simulink model "Model_Dimitri"  (R2023b)
settings: Solver=ode23tb  StartTime=0.0  StopTime=1.5  FixedStep=1e-6  MaxStep=1/50/100  RelTol=1e-3
values from neighbouring files (symbols this model uses):
  B = 0.0129    [PARAMETERS_MODEL_GR2.m]    (also in Parameters.m; Parameters_Chloe.m)
  C_dc = 15e-3    (= 0.015)    [PARAMETERS_MODEL_GR2.m]    (also in Parameters.m; Parameters_Chloe.m)
  f_grid = 50    [PARAMETERS_MODEL_GR2.m]    (also in Parameters.m; Parameters_Chloe.m)
  f_r = 50    [PARAMETERS_MODEL_GR2.m]    (also in Parameters.m; Parameters_Chloe.m)
  J = 0.2799    [PARAMETERS_MODEL_GR2.m]    (also in Parameters.m; Parameters_Chloe.m)
  L_grid = 1.5e-6    (= 1.5e-06)    [PARAMETERS_MODEL_GR2.m]    (also in Parameters.m = 1e-12; Parameters_Chloe.m = 2e-05)
  L_lr = 1.8e-3    (= 0.0018)    [PARAMETERS_MODEL_GR2.m]    (also in Parameters.m = 1.8; Parameters_Chloe.m)
  L_ls = 1.8e-3    (= 0.0018)    [PARAMETERS_MODEL_GR2.m]    (also in Parameters.m = 1.8; Parameters_Chloe.m)
  L_rectif = 10e-3    (= 0.01)    [PARAMETERS_MODEL_GR2.m]    (also in Parameters.m; Parameters_Chloe.m)
  P = 4    [PARAMETERS_MODEL_GR2.m]    (also in Parameters.m; Parameters_Chloe.m)
  P_r = 19e3    (= 19000)    [PARAMETERS_MODEL_GR2.m]    (also in Parameters.m; Parameters_Chloe.m)
  R_grid = 0.005    [PARAMETERS_MODEL_GR2.m]    (also in Parameters.m = 0.001; Parameters_Chloe.m = 0.2)
  R_r = 0.1091    [PARAMETERS_MODEL_GR2.m]    (also in Parameters.m; Parameters_Chloe.m)
  R_s = 0.0629    [PARAMETERS_MODEL_GR2.m]    (also in Parameters.m; Parameters_Chloe.m)
  U_ac = 380    [PARAMETERS_MODEL_GR2.m]    (also in Parameters.m; Parameters_Chloe.m)
  V_r = 400    [PARAMETERS_MODEL_GR2.m]    (also in Parameters.m; Parameters_Chloe.m)
libraries: spsSeriesRLCBranchLib x10, spsDiodeLib x6, spsMosfetLib x6, spsVoltageMeasurementLib x5, spsThreePhaseVIMeasurementLib x4, spsACVoltageSourceLib x3, spsThreePhaseTransformerTwoWindingsLib x2, spsAsynchronousMachinepuUnitsLib x2, spsCurrentMeasurementLib x2, spsGroundLib x1, spsThreePhaseSourceLib x1, spsTriangleGeneratorLib x1
settings Model: Creator=dimit  LastModifiedBy=dimit

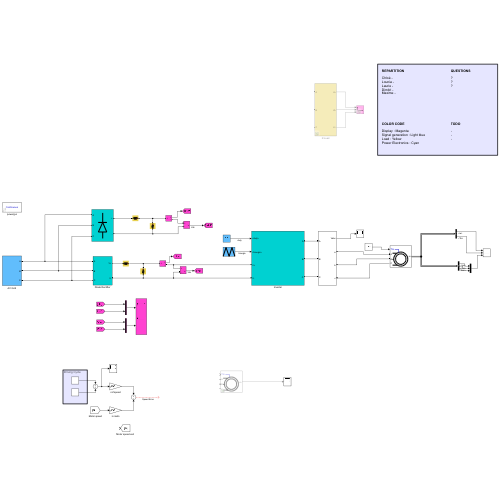
[thumbnail: Simulink's stored preview of the top-level diagram]
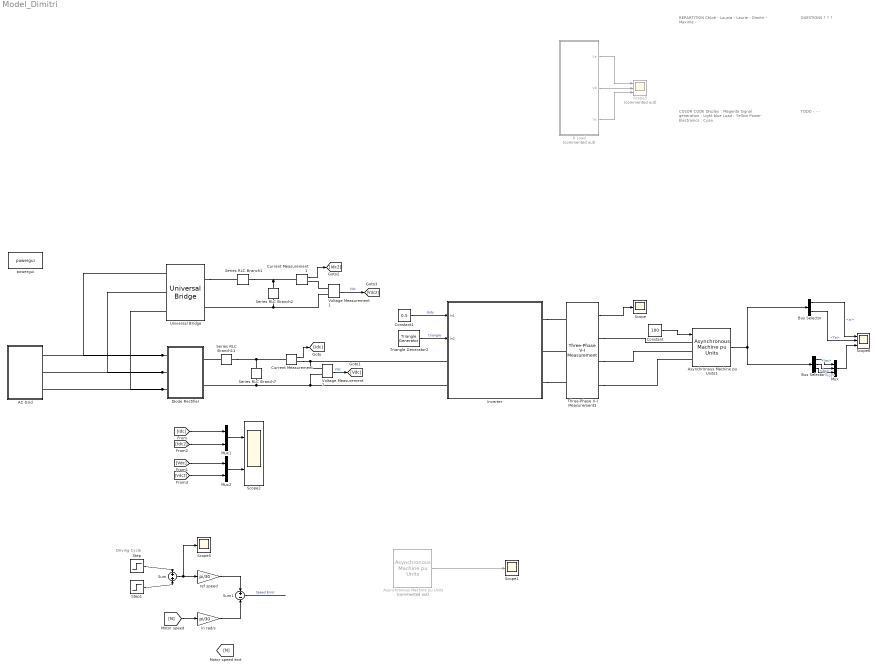
== system Model_Dimitri ==
  note: COLOR CODE
      |
      | Display : Magenta
      | Signal generation : Light blue
      | Load : Yellow
      | Power Electronics : Cyan
  note: Driving Cycle
  note: QUESTIONS
      |
      | ?
      | ?
      | ?
  note: TODO
      |
      | -
      | -
      | -
  note: REPARTITION
      |
      | Chloé -
      | Lounia -
      | Laurie -
      | Dimitri -
      | Maxime -
  AC Grid : Subsystem
  Asynchronous Machine pu Units : spsAsynchronousMachinepuUnitsLib/Asynchronous Machine pu Units  Commented=on  RotorType=Squirrel-cage  PresetModel=No  MechanicalLoad=Torque Tm  ShowDetailedParameters=on  ReferenceFrame=Rotor  Units=pu  MeasurementBus=on  NominalParameters=[3730 460 60]  VoltageRatio=1  Stator=[R_s L_ls]  Rotor=[R_r L_lr]  Cage1=[0.01909 0.0397]  Cage2=[0.01909 0.0397]  Lm=L_m  Mechanical=[J B P]  PolePairs=2  InitialConditions="[ 1,0   0,0,0   0,0,0 ]"  SimulateSaturation=off  Saturation="[0.212,0.4201,0.8125,1.0979,1.4799,2.2457,3.2586,4.5763,6.4763 ;   0.5,0.7,0.9,1,1.1,1.2 ,1.3,1.4,1.5]"  LoadFlowParameters=0  TsPowergui=0  TsBlock=-1  IterativeModel=Trapezoidal non iterative  IterativeDiscreteModel=Trapezoidal non iterative  Pmec=0
      settings: LibrarySourceBlock=|
      | sps_lib/Electrical Machines/Asynchronous Machine
      | pu Units
  Asynchronous Machine pu Units1 : spsAsynchronousMachinepuUnitsLib/Asynchronous Machine pu Units  RotorType=Squirrel-cage  PresetModel=No  MechanicalLoad=Torque Tm  ShowDetailedParameters=on  ReferenceFrame=Rotor  Units=pu  MeasurementBus=on  NominalParameters=[P_r V_r f_r]  VoltageRatio=1  Stator=[R_s L_ls]  Rotor=[R_r L_lr]  Cage1=[0.01909 0.0397]  Cage2=[0.01909 0.0397]  Lm=L_m  Mechanical=[J B P]  PolePairs=2  InitialConditions="[ 1,0   0,0,0   0,0,0]"  SimulateSaturation=off  Saturation="[0.212,0.4201,0.8125,1.0979,1.4799,2.2457,3.2586,4.5763,6.4763 ;   0.5,0.7,0.9,1,1.1,1.2 ,1.3,1.4,1.5]"  LoadFlowParameters=0  TsPowergui=0  TsBlock=-1  IterativeModel=Trapezoidal non iterative  IterativeDiscreteModel=Trapezoidal non iterative  Pmec=0
      settings: LibrarySourceBlock=|
      | sps_lib/Electrical Machines/Asynchronous Machine
      | pu Units
  Bus Selector : BusSelector  OutputSignals=w,Te
  Bus Selector1 : BusSelector  OutputSignals=ias,ibs,ics
  Constant : Constant  Value=100
  Constant1 : Constant  Value=0.5
  Current Measurement : spsCurrentMeasurementLib/Current Measurement  PhasorSimulation=off  OutputType=Complex  PSBequivalent=0
  Current Measurement1 : spsCurrentMeasurementLib/Current Measurement  PhasorSimulation=off  OutputType=Complex  PSBequivalent=0
  Diode Rectifier : Subsystem
  Inverter : Subsystem
  Mux : Mux  Inputs=3
  Mux1 : Mux  Inputs=2
  Mux2 : Mux  Inputs=2
  R Load : Subsystem  Commented=on
  Scope : Scope
  Scope1 : Scope
  Scope2 : Scope  NumInputPorts=2
  Scope3 : Scope  Commented=on  NumInputPorts=3
  Scope5 : Scope
  Scope6 : Scope  NumInputPorts=3
  Series RLC Branch1 : spsSeriesRLCBranchLib/Series RLC Branch  LConnTagsString=__new0  RConnTagsString=__new0  BranchType=L  Resistance=1  Inductance=L_rectif  SetiL0=off  InitialCurrent=0  Capacitance=15e-6  Setx0=off  InitialVoltage=0  Measurements=None
  Series RLC Branch11 : spsSeriesRLCBranchLib/Series RLC Branch  LConnTagsString=__new0  RConnTagsString=__new0  BranchType=L  Resistance=1  Inductance=L_rectif  SetiL0=off  InitialCurrent=0  Capacitance=15e-6  Setx0=off  InitialVoltage=0  Measurements=None
  Series RLC Branch2 : spsSeriesRLCBranchLib/Series RLC Branch  LConnTagsString=__new0  RConnTagsString=__new0  BranchType=C  Resistance=1  Inductance=1e-3  SetiL0=off  InitialCurrent=0  Capacitance=C_dc  Setx0=off  InitialVoltage=0  Measurements=None
  Series RLC Branch7 : spsSeriesRLCBranchLib/Series RLC Branch  LConnTagsString=__new0  RConnTagsString=__new0  BranchType=C  Resistance=1  Inductance=1e-3  SetiL0=off  InitialCurrent=0  Capacitance=C_dc  Setx0=off  InitialVoltage=0  Measurements=None
  Step : Step  Time=0.1  After=1200  SampleTime=0
  Step1 : Step  Time=1.7  After=-1200  SampleTime=0
  Sum : Sum  Inputs=+|+
  Sum1 : Sum  Inputs=+|-
  Three-Phase V-I Measurement1 : spsThreePhaseVIMeasurementLib/Three-Phase V-I Measurement  VoltageMeasurement=phase-to-phase  SetLabelV=off  LabelV=Vabc  Vpu=off  VpuLL=off  CurrentMeasurement=no  SetLabelI=off  LabelI=Iabc  Ipu=off  Pbase=100e6  Vbase=500e3  OutputType=Complex  PhasorSimulation=off  PSBequivalent=0
  Triangle Generator2 : spsTriangleGeneratorLib/Triangle Generator  Freq=f_r*39  Phase=0  Ts=0
  Universal Bridge : spsUniversalBridgeLib/Universal Bridge  Arms=3  SnubberResistance=R_snubber  SnubberCapacitance=C_snubber  Device=Diodes  Ron=R_on  Lon=0  ForwardVoltages="[  0  0  ]"  ForwardVoltage=V_f  GTOparameters=[ 10e-6 , 20e-6 ]  IGBTparameters=[ 1e-6 , 2e-6 ]  Measurements=None  Measurements_2=None  converterType=Rectifier
  Voltage Measurement1 : spsVoltageMeasurementLib/Voltage Measurement  PhasorSimulation=off  OutputType=Complex  PSBequivalent=0
  Voltage Measurement7 : spsVoltageMeasurementLib/Voltage Measurement  PhasorSimulation=off  OutputType=Complex  PSBequivalent=0
  in rad/s : Gain  Gain=pi/30
  powergui : sps_lib/powergui  Priority=1  SimulationMode=Continuous  SampleTime=1e-6  frequency=60  Iterations=50  frequencyindice=50  Pbase=100e6  ErrMax=1e-4  UnitsV=kV  UnitsW=MW  buscounter=0  FunctionMessages=off  echomessages=off  EnableUseOfTLC=off  CurrentSourceSwitches=off  DisableSnubberDevices=off  DisableRonSwitches=off  DisableVfSwitches=off  DisplayEquations=off  AutomaticDiscreteSolvers=off  SolverType=Tustin/Backward Euler (TBE)  Interpol=off  ExternalGateDelay=off  methode=off  Ts=100  x0status=blocks  SPID=on  SwTol=0  HookPort=off  NonlinearTolerance=1e-4  nMaxIteration=100  ContinueOnMaxIteration=off  RestoreLinks=warning  ResistiveCurrentMeasurement=off  Frange=[0:2:500]  Ylog=off  Xlog=on  ShowGrid=off  save=off  variable=ZData  structure=0  ZoomFFT=off  StartTime=0.0  cycles=1  DisplayStyle=1  fundamental=60  FreqAxis=off  MaxFrequency=1000  frequencyindicesteady=1  RmsSteady=1  display=off
  ref speed : Gain  Gain=pi/30
  wires:
  Triangle Generator2/1 -> Inverter/2(In2)  "triangle"
  Constant1/1 -> Inverter/1(In1)  "duty"
  Sum1/1 -> ?  "Speed Error"
  [N] -> in rad/s/1
  Step1/1 -> Sum/2
  Sum/1 -> ref speed/1, Scope5/1
  ref speed/1 -> Sum1/1
  in rad/s/1 -> Sum1/2
  Step/1 -> Sum/1
  Asynchronous Machine pu Units/1 -> Scope1/1
  R Load/1(Va) -> Scope3/1
  R Load/2(Vb) -> Scope3/2
  R Load/3(Vc) -> Scope3/3
  Constant/1 -> Asynchronous Machine pu Units1/1
  Asynchronous Machine pu Units1/1 -> Bus Selector/1, Bus Selector1/1
  Bus Selector1/1 -> Mux/1  "<ias>"
  Bus Selector1/2 -> Mux/2  "<ibs>"
  Bus Selector1/3 -> Mux/3  "<ics>"
  Mux/1 -> Scope6/3
  Bus Selector/1 -> Scope6/1  "<w>"
  Bus Selector/2 -> Scope6/2  "<Te>"
  Three-Phase V-I Measurement1/1 -> Scope/1
  Current Measurement/1 -> [Idc]
  Voltage Measurement7/1 -> [Vdc]  "Vdc"
  Current Measurement1/1 -> [Idc2]
  Voltage Measurement1/1 -> [Vdc2]  "Vdc"
  [Idc] -> Mux1/1
  [Vdc] -> Mux2/1
  [Vdc2] -> Mux2/2
  [Idc2] -> Mux1/2
  Mux1/1 -> Scope2/1
  Mux2/1 -> Scope2/2
  connections:
  Diode Rectifier/LConn1 -- Universal Bridge/LConn1 -- AC Grid/LConn1
  Diode Rectifier/LConn2 -- Universal Bridge/LConn2 -- AC Grid/LConn2
  Diode Rectifier/LConn3 -- Universal Bridge/LConn3 -- AC Grid/LConn3
  Inverter/LConn2 -- Diode Rectifier/RConn2 -- Series RLC Branch7/RConn1 -- Voltage Measurement7/LConn2
  Voltage Measurement7/LConn1 -- Inverter/LConn1 -- Current Measurement/RConn1
  Series RLC Branch11/RConn1 -- Diode Rectifier/RConn1
  Series RLC Branch11/LConn1 -- Current Measurement/LConn1 -- Series RLC Branch7/LConn1
  Three-Phase V-I Measurement1/LConn2 -- Inverter/RConn2
  Inverter/RConn1 -- Three-Phase V-I Measurement1/LConn1
  Inverter/RConn3 -- Three-Phase V-I Measurement1/LConn3
  Three-Phase V-I Measurement1/RConn1 -- Asynchronous Machine pu Units1/LConn1
  Three-Phase V-I Measurement1/RConn2 -- Asynchronous Machine pu Units1/LConn2
  Three-Phase V-I Measurement1/RConn3 -- Asynchronous Machine pu Units1/LConn3
  Voltage Measurement1/LConn1 -- Current Measurement1/RConn1
  Series RLC Branch2/LConn1 -- Series RLC Branch1/LConn1 -- Current Measurement1/LConn1
  Series RLC Branch2/RConn1 -- Voltage Measurement1/LConn2 -- Universal Bridge/RConn2
  Universal Bridge/RConn1 -- Series RLC Branch1/RConn1

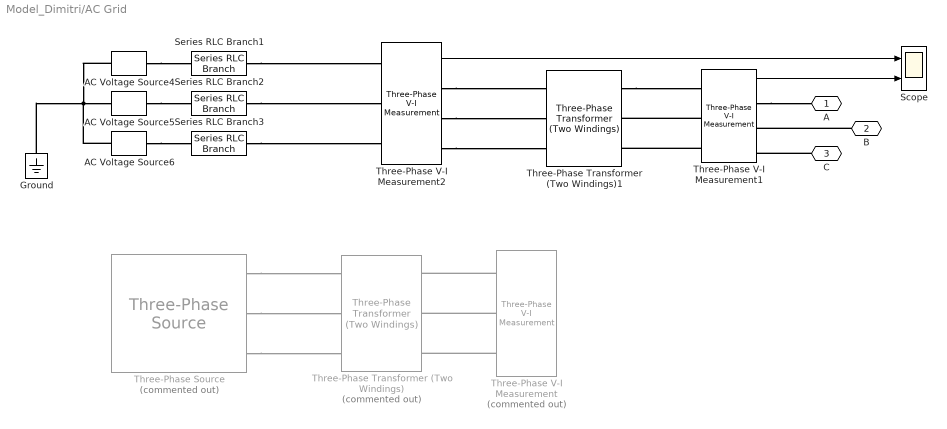
== system Model_Dimitri/AC Grid ==
  AC Voltage Source4 : spsACVoltageSourceLib/AC Voltage Source  Amplitude=U_ac/sqrt(3)*sqrt(2)  Phase=0  Frequency=f_grid  SampleTime=0  Measurements=None  BusType=swing  Pref=10e3  Qref=0  Qmin=-inf  Qmax=+inf
  AC Voltage Source5 : spsACVoltageSourceLib/AC Voltage Source  Amplitude=U_ac/sqrt(3)*sqrt(2)  Phase=-120  Frequency=f_grid  SampleTime=0  Measurements=None  BusType=swing  Pref=10e3  Qref=0  Qmin=-inf  Qmax=+inf
  AC Voltage Source6 : spsACVoltageSourceLib/AC Voltage Source  Amplitude=U_ac/sqrt(3)*sqrt(2)  Phase=120  Frequency=f_grid  SampleTime=0  Measurements=None  BusType=swing  Pref=10e3  Qref=0  Qmin=-inf  Qmax=+inf
  Ground : spsGroundLib/Ground  LConnTagsString=a
  Scope : Scope  NumInputPorts=2
  Series RLC Branch1 : spsSeriesRLCBranchLib/Series RLC Branch  LConnTagsString=__new0  RConnTagsString=__new0  BranchType=RL  Resistance=R_grid  Inductance=L_grid  SetiL0=off  InitialCurrent=0  Capacitance=15e-6  Setx0=off  InitialVoltage=0  Measurements=None
  Series RLC Branch2 : spsSeriesRLCBranchLib/Series RLC Branch  LConnTagsString=__new0  RConnTagsString=__new0  BranchType=RL  Resistance=R_grid  Inductance=L_grid  SetiL0=off  InitialCurrent=0  Capacitance=15e-6  Setx0=off  InitialVoltage=0  Measurements=None
  Series RLC Branch3 : spsSeriesRLCBranchLib/Series RLC Branch  LConnTagsString=__new0  RConnTagsString=__new0  BranchType=RL  Resistance=R_grid  Inductance=L_grid  SetiL0=off  InitialCurrent=0  Capacitance=15e-6  Setx0=off  InitialVoltage=0  Measurements=None
  Three-Phase Transformer (Two Windings) : spsThreePhaseTransformerTwoWindingsLib/Three-Phase Transformer (Two Windings)  Commented=on  Winding1Connection=Y  Winding2Connection=Y  CoreType=Three single-phase transformers  SetSaturation=off  Hysteresis=off  DataFile='hysteresis'  SetInitialFlux=off  Measurements=None  UNITS=pu  NominalPower=[ 20e3 , 50 ]  Winding1=[ 380 , 0.002 , 0.08 ]  Winding2=[ 380 , 0.002 , 0.08 ]  Rm=500  Lm=500  L0=0.5  Saturation=[ 0,0 ; 0.0024,1.2 ; 1.0,1.52 ]  InitialFluxes=[ 0.8 , -0.8 , 0.7 ]  BreakLoop=off  DiscreteSolver=Trapezoidal iterative  DataType=off  TransfoNumber=1
  Three-Phase Transformer (Two Windings)1 : spsThreePhaseTransformerTwoWindingsLib/Three-Phase Transformer (Two Windings)  Winding1Connection=Y  Winding2Connection=Y  CoreType=Three single-phase transformers  SetSaturation=off  Hysteresis=off  DataFile='hysteresis'  SetInitialFlux=off  Measurements=None  UNITS=pu  NominalPower=[ 20e3 , 50 ]  Winding1=[ 380 , 0.002 , 0.08 ]  Winding2=[ 380 , 0.002 , 0.08 ]  Rm=500  Lm=500  L0=0.5  Saturation=[ 0,0 ; 0.0024,1.2 ; 1.0,1.52 ]  InitialFluxes=[ 0.8 , -0.8 , 0.7 ]  BreakLoop=off  DiscreteSolver=Trapezoidal iterative  DataType=off  TransfoNumber=1
  Three-Phase V-I Measurement : spsThreePhaseVIMeasurementLib/Three-Phase V-I Measurement  Commented=on  VoltageMeasurement=phase-to-phase  SetLabelV=off  LabelV=Vabc  Vpu=off  VpuLL=off  CurrentMeasurement=no  SetLabelI=off  LabelI=Iabc  Ipu=off  Pbase=100e6  Vbase=500e3  OutputType=Complex  PhasorSimulation=off  PSBequivalent=0
  Three-Phase V-I Measurement1 : spsThreePhaseVIMeasurementLib/Three-Phase V-I Measurement  VoltageMeasurement=phase-to-phase  SetLabelV=off  LabelV=Vabc  Vpu=off  VpuLL=off  CurrentMeasurement=no  SetLabelI=off  LabelI=Iabc  Ipu=off  Pbase=100e6  Vbase=500e3  OutputType=Complex  PhasorSimulation=off  PSBequivalent=0
  Three-Phase V-I Measurement2 : spsThreePhaseVIMeasurementLib/Three-Phase V-I Measurement  VoltageMeasurement=phase-to-phase  SetLabelV=off  LabelV=Vabc  Vpu=off  VpuLL=off  CurrentMeasurement=no  SetLabelI=off  LabelI=Iabc  Ipu=off  Pbase=100e6  Vbase=500e3  OutputType=Complex  PhasorSimulation=off  PSBequivalent=0
  Three-Phase Source : spsThreePhaseSourceLib/Three-Phase Source  Commented=on  InternalConnection=Yg  VoltagePhases=off  Voltage=U_ac  PhaseAngle=0  Voltage_phases=[25e3 25e3 25e3]/sqrt(3)  PhaseAngles_phases=[0 -120 +120]  Frequency=f_grid  NonIdealSource=on  SpecifyImpedance=off  Resistance=R_grid  Inductance=L_grid  ShortCircuitLevel=100e6  BaseVoltage=U_ac  XRratio=7  BusType=swing  Pref=10e3  Qref=0  Prefabc=[10e3, 10e3, 10e3]  Qrefabc=[0, 0, 0]  Qmin=-inf  Qmax=inf
  A : PMIOPort  Side=Left
  B : PMIOPort  Port=2  Side=Left
  C : PMIOPort  Port=3  Side=Left
  wires:
  Three-Phase V-I Measurement1/1 -> Scope/2
  Three-Phase V-I Measurement2/1 -> Scope/1
  connections:
  AC Voltage Source6/LConn1 -- Ground/LConn1 -- AC Voltage Source5/LConn1 -- AC Voltage Source4/LConn1
  AC Voltage Source5/RConn1 -- Series RLC Branch2/RConn1
  AC Voltage Source6/RConn1 -- Series RLC Branch3/RConn1
  Three-Phase Source/RConn1 -- Three-Phase Transformer (Two Windings)/LConn1
  Three-Phase Source/RConn2 -- Three-Phase Transformer (Two Windings)/LConn2
  Three-Phase Source/RConn3 -- Three-Phase Transformer (Two Windings)/LConn3
  Three-Phase V-I Measurement/LConn1 -- Three-Phase Transformer (Two Windings)/RConn1
  Three-Phase V-I Measurement/LConn2 -- Three-Phase Transformer (Two Windings)/RConn2
  Three-Phase V-I Measurement/LConn3 -- Three-Phase Transformer (Two Windings)/RConn3
  Three-Phase Transformer (Two Windings)1/RConn1 -- Three-Phase V-I Measurement1/LConn1
  Three-Phase V-I Measurement1/LConn2 -- Three-Phase Transformer (Two Windings)1/RConn2
  Three-Phase V-I Measurement1/LConn3 -- Three-Phase Transformer (Two Windings)1/RConn3
  AC Voltage Source4/RConn1 -- Series RLC Branch1/RConn1
  Three-Phase V-I Measurement1/RConn1 -- A/RConn1
  C/RConn1 -- Three-Phase V-I Measurement1/RConn3
  B/RConn1 -- Three-Phase V-I Measurement1/RConn2
  Series RLC Branch1/LConn1 -- Three-Phase V-I Measurement2/LConn1
  Series RLC Branch2/LConn1 -- Three-Phase V-I Measurement2/LConn2
  Series RLC Branch3/LConn1 -- Three-Phase V-I Measurement2/LConn3
  Three-Phase V-I Measurement2/RConn1 -- Three-Phase Transformer (Two Windings)1/LConn1
  Three-Phase V-I Measurement2/RConn2 -- Three-Phase Transformer (Two Windings)1/LConn2
  Three-Phase V-I Measurement2/RConn3 -- Three-Phase Transformer (Two Windings)1/LConn3

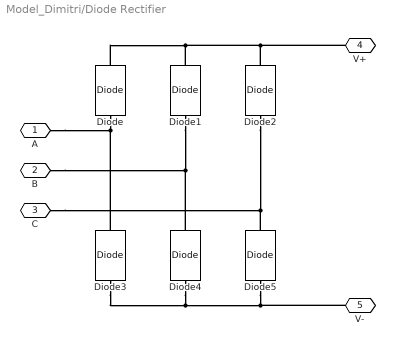
== system Model_Dimitri/Diode Rectifier ==
  Diode{,1..5} (6 alike) : spsDiodeLib/Diode  Ron=R_on  Lon=0  Vf=V_f  IC=0  UseSnubber=0  Rs=R_snubber  Cs=C_snubber  Measurements=off
  A : PMIOPort  Side=Left
  B : PMIOPort  Port=2  Side=Left
  C : PMIOPort  Port=3  Side=Left
  V+ : PMIOPort  Port=4  Side=Right
  V- : PMIOPort  Port=5  Side=Right
  connections:
  B/RConn1 -- Diode1/LConn1 -- Diode4/RConn1
  Diode4/LConn1 -- Diode3/LConn1 -- Diode5/LConn1 -- V-/RConn1
  C/RConn1 -- Diode2/LConn1 -- Diode5/RConn1
  Diode/LConn1 -- Diode3/RConn1 -- A/RConn1
  Diode/RConn1 -- V+/RConn1 -- Diode2/RConn1 -- Diode1/RConn1

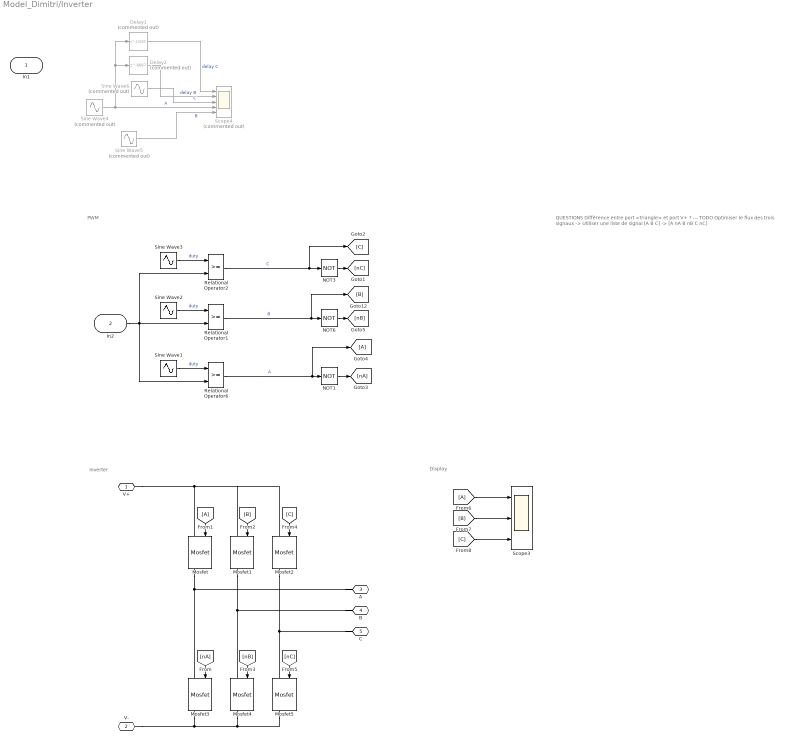
== system Model_Dimitri/Inverter ==
  note: Display
  note: PWM
  note: QUESTIONS
      |
      | Différence entre port <triangle> et port V+ ?
      |
      | ---
      |
      | TODO
      |
      | Optimiser le flux des trois signaux -> Utiliser une liste de signal [A B C] -> [A nA B nB C nC]
  note: Inverter
  In1 : Inport
  In2 : Inport  Port=2
  Delay1 : Delay  Commented=on  DelayLength=13333
  Delay2 : Delay  Commented=on  DelayLength=6667
  From1 : From
  From6 : From
  Goto4 : Goto
  Mosfet{,1..5} (6 alike) : spsMosfetLib/Mosfet  Ron=R_on_fet  Lon=0  Rd=R_d  Vfd=V_f_inv  IC=0  Rs=R_snub_inv  Cs=C_snub_inv  Measurements=on
  NOT1 : Logic  Operator=NOT  AllPortsSameDT=off  OutDataTypeStr=boolean
  NOT3 : Logic  Operator=NOT  AllPortsSameDT=off  OutDataTypeStr=boolean
  NOT6 : Logic  Operator=NOT  AllPortsSameDT=off  OutDataTypeStr=boolean
  Relational Operator1 : RelationalOperator  OutDataTypeStr=boolean  RndMeth=Simplest  InputSameDT=off
  Relational Operator2 : RelationalOperator  OutDataTypeStr=boolean  RndMeth=Simplest  InputSameDT=off
  Relational Operator6 : RelationalOperator  OutDataTypeStr=boolean  RndMeth=Simplest  InputSameDT=off
  Scope3 : Scope  NumInputPorts=3
  Scope4 : Scope  Commented=on  NumInputPorts=5
  Sine Wave1 : Sin  Frequency=2*pi*50  SampleTime=0
  Sine Wave2 : Sin  Frequency=2*pi*50  Phase=4*pi/3  SampleTime=0
  Sine Wave3 : Sin  Frequency=2*pi*50  Phase=2*pi/3  SampleTime=0
  Sine Wave4 : Sin  Commented=on  Frequency=2*pi*50  SampleTime=0
  Sine Wave5 : Sin  Commented=on  Frequency=2*pi*50  Phase=4*pi/3  SampleTime=0
  Sine Wave6 : Sin  Commented=on  Frequency=2*pi*50  Phase=2*pi/3  SampleTime=0
  V+ : PMIOPort  Side=Left
  V- : PMIOPort  Port=2  Side=Left
  A : PMIOPort  Port=3  Side=Right
  B : PMIOPort  Port=4  Side=Right
  C : PMIOPort  Port=5  Side=Right
  wires:
  [nA] -> Mosfet3/1
  [C] -> Mosfet2/1
  [nB] -> Mosfet4/1
  From1/1 -> Mosfet/1
  [nC] -> Mosfet5/1
  Sine Wave3/1 -> Relational Operator2/1  "duty"
  Relational Operator1/1 -> [B], NOT6/1  "B"
  Relational Operator6/1 -> Goto4/1, NOT1/1  "A"
  Sine Wave2/1 -> Relational Operator1/1  "duty"
  Sine Wave1/1 -> Relational Operator6/1  "duty"
  Relational Operator2/1 -> [C], NOT3/1  "C"
  NOT1/1 -> [nA]
  NOT6/1 -> [nB]
  NOT3/1 -> [nC]
  Sine Wave4/1 -> Delay2/1, Delay1/1, Scope4/4  "A"
  Sine Wave5/1 -> Scope4/5  "B"
  Sine Wave6/1 -> Scope4/3  "C"
  Delay2/1 -> Scope4/2  "delay B"
  Delay1/1 -> Scope4/1  "delay C"
  In2/1 -> Relational Operator2/2, Relational Operator6/2, Relational Operator1/2
  From6/1 -> Scope3/1
  [B] -> Scope3/2
  [C] -> Scope3/3
  [B] -> Mosfet1/1
  connections:
  C/RConn1 -- Mosfet5/LConn1 -- Mosfet2/RConn1
  Mosfet2/LConn1 -- Mosfet1/LConn1 -- Mosfet/LConn1 -- V+/RConn1
  V-/RConn1 -- Mosfet3/RConn1 -- Mosfet5/RConn1 -- Mosfet4/RConn1
  B/RConn1 -- Mosfet4/LConn1 -- Mosfet1/RConn1
  A/RConn1 -- Mosfet3/LConn1 -- Mosfet/RConn1

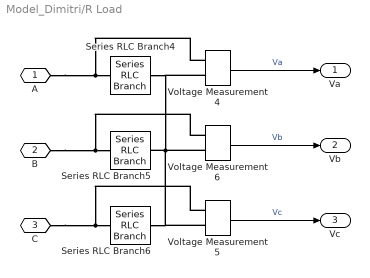
== system Model_Dimitri/R Load ==
  Series RLC Branch4 : spsSeriesRLCBranchLib/Series RLC Branch  LConnTagsString=__new0  RConnTagsString=__new0  BranchType=R  Resistance=1  Inductance=0  SetiL0=off  InitialCurrent=0  Capacitance=0  Setx0=off  InitialVoltage=0  Measurements=None
  Series RLC Branch5 : spsSeriesRLCBranchLib/Series RLC Branch  LConnTagsString=__new0  RConnTagsString=__new0  BranchType=R  Resistance=1  Inductance=0  SetiL0=off  InitialCurrent=0  Capacitance=0  Setx0=off  InitialVoltage=0  Measurements=None
  Series RLC Branch6 : spsSeriesRLCBranchLib/Series RLC Branch  LConnTagsString=__new0  RConnTagsString=__new0  BranchType=R  Resistance=1  Inductance=0  SetiL0=off  InitialCurrent=0  Capacitance=0  Setx0=off  InitialVoltage=0  Measurements=None
  Voltage Measurement4 : spsVoltageMeasurementLib/Voltage Measurement  PhasorSimulation=off  OutputType=Complex  PSBequivalent=0
  Voltage Measurement5 : spsVoltageMeasurementLib/Voltage Measurement  PhasorSimulation=off  OutputType=Complex  PSBequivalent=0
  Voltage Measurement6 : spsVoltageMeasurementLib/Voltage Measurement  PhasorSimulation=off  OutputType=Complex  PSBequivalent=0
  A : PMIOPort  Side=Left
  B : PMIOPort  Port=2  Side=Left
  C : PMIOPort  Port=3  Side=Left
  Va : Outport
  Vb : Outport  Port=2
  Vc : Outport  Port=3
  wires:
  Voltage Measurement5/1 -> Vc/1  "Vc"
  Voltage Measurement4/1 -> Va/1  "Va"
  Voltage Measurement6/1 -> Vb/1  "Vb"
  connections:
  Series RLC Branch5/LConn1 -- Voltage Measurement4/LConn2 -- Series RLC Branch4/LConn1 -- Voltage Measurement6/LConn2 -- Series RLC Branch6/LConn1 -- Voltage Measurement5/LConn2
  Series RLC Branch4/RConn1 -- A/RConn1 -- Voltage Measurement4/LConn1
  Series RLC Branch6/RConn1 -- C/RConn1 -- Voltage Measurement5/LConn1
  Series RLC Branch5/RConn1 -- B/RConn1 -- Voltage Measurement6/LConn1
